simulink model "REDCS_Pipeline_IntermediateModel_FSU_29APR2022"  (R2022a)
settings: Solver=VariableStepAuto  StartTime=0.0  StopTime=3600  RelTol=1e-3
values from neighbouring files (symbols this model uses):
  Ac = (pi/4)*0.6096^2    (= 0.29186350796)    [REDCS_IntermediateModel_Parameters_29APR2022.m]
  B1 = 45    [REDCS_IntermediateModel_Parameters_29APR2022.m]
  CLOSED = 0    [REDCS_IntermediateModel_Parameters_29APR2022.m]
  EP020 = 21.9    [REDCS_IntermediateModel_Parameters_29APR2022.m]
  EP022 = 13.1    [REDCS_IntermediateModel_Parameters_29APR2022.m]
  EP024 = 54.2    [REDCS_IntermediateModel_Parameters_29APR2022.m]
  EP026 = 13.4    [REDCS_IntermediateModel_Parameters_29APR2022.m]
  EP028 = 0.5    [REDCS_IntermediateModel_Parameters_29APR2022.m]
  gamma = 1.2    [REDCS_IntermediateModel_Parameters_29APR2022.m]
  J = 5    [REDCS_IntermediateModel_Parameters_29APR2022.m]
  kf = 0.05    [REDCS_IntermediateModel_Parameters_29APR2022.m]
  Lc = 20    [REDCS_IntermediateModel_Parameters_29APR2022.m]
  OPEN = 1    [REDCS_IntermediateModel_Parameters_29APR2022.m]
  r1 = 0.05    [REDCS_IntermediateModel_Parameters_29APR2022.m]
  r2 = 0.325    [REDCS_IntermediateModel_Parameters_29APR2022.m]
  sigma = 0.90    (= 0.9)    [REDCS_IntermediateModel_Parameters_29APR2022.m]
  ValveThresh = 0.001    [REDCS_IntermediateModel_Parameters_29APR2022.m]
  ZR2000 = OPEN    (= 1)    [REDCS_IntermediateModel_Parameters_29APR2022.m]
  ZR2110 = CLOSED    (= 0)    [REDCS_IntermediateModel_Parameters_29APR2022.m]
  ZR2400 = OPEN    (= 1)    [REDCS_IntermediateModel_Parameters_29APR2022.m]
  ZR2401 = 100*OPEN    (= 100)    [REDCS_IntermediateModel_Parameters_29APR2022.m]
  ZR2510 = CLOSED    (= 0)    [REDCS_IntermediateModel_Parameters_29APR2022.m]
  ZR2600 = OPEN    (= 1)    [REDCS_IntermediateModel_Parameters_29APR2022.m]
  ZR2601 = 100*OPEN    (= 100)    [REDCS_IntermediateModel_Parameters_29APR2022.m]
  ZR2700 = OPEN    (= 1)    [REDCS_IntermediateModel_Parameters_29APR2022.m]
  ZR2701 = 100*OPEN    (= 100)    [REDCS_IntermediateModel_Parameters_29APR2022.m]
  ZR2800 = OPEN    (= 1)    [REDCS_IntermediateModel_Parameters_29APR2022.m]
  ZR2801 = 100*OPEN    (= 100)    [REDCS_IntermediateModel_Parameters_29APR2022.m]
  ZR2900 = OPEN    (= 1)    [REDCS_IntermediateModel_Parameters_29APR2022.m]
  ZR2901 = 100*OPEN    (= 100)    [REDCS_IntermediateModel_Parameters_29APR2022.m]
  ZR3900 = OPEN    (= 1)    [REDCS_IntermediateModel_Parameters_29APR2022.m]
  ZR4500 = OPEN    (= 1)    [REDCS_IntermediateModel_Parameters_29APR2022.m]
  ZR5600 = OPEN    (= 1)    [REDCS_IntermediateModel_Parameters_29APR2022.m]
  ZR7800 = CLOSED    (= 0)    [REDCS_IntermediateModel_Parameters_29APR2022.m]
undefined symbols (not defined in the file or in its folder): cotd, LEG_DEMAND_10A, LEG_DEMAND_3A, magnitude
libraries: fl_lib x170, nesl_utility x109, simulink x12, slpidlib x4
(part 2 of 4)

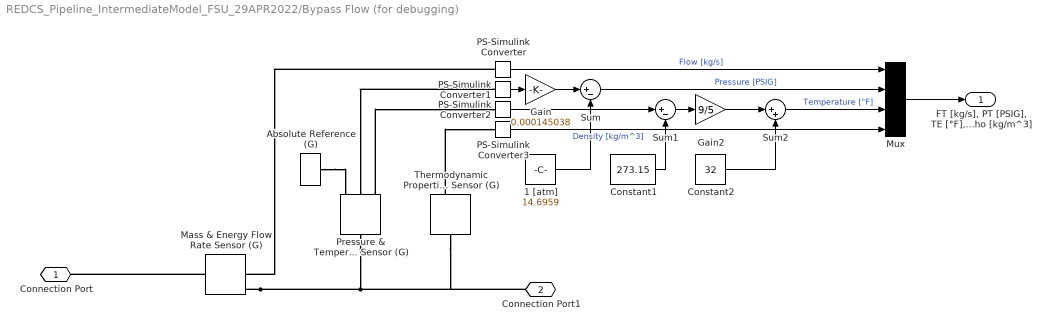
== system REDCS_Pipeline_IntermediateModel_FSU_29APR2022/Bypass Flow (for debugging) ==
  1 [atm] : Constant  Value=14.6959
  Absolute Reference (G) : fl_lib/Gas/Elements/Absolute Reference (G)
      settings: SourceProductBaseCode=PW,SS,VE  InternalSimscapePortConfiguration="{\"Bottom\":[],\"Left\":[{\"id\":\"A\",\"label\":\"\",\"type\":\"foundation.gas.gas\"}],\"Right\":[],\"Top\":[]}"
  Constant1 : Constant  Value=273.15
  Constant2 : Constant  Value=32
  Gain : Gain  Gain=0.000145038
  Gain2 : Gain  Gain=9/5
  Mass & Energy Flow Rate Sensor (G) : fl_lib/Gas/Sensors/Mass & Energy Flow Rate Sensor (G)
      settings: SourceProductBaseCode=PW,SS,VE  InternalSimscapePortConfiguration="{\"Bottom\":[],\"Left\":[{\"id\":\"A\",\"label\":\"A\",\"type\":\"foundation.gas.gas\"}],\"Right\":[{\"id\":\"B\",\"label\":\"B\",\"type\":\"foundation.gas.gas\"},{\"id\":\"M\",\"label\":\"M\",\"type\":\"output\"},{\"id\":\"PHI\",\"label\":\"Phi\",\"type\":\"output\"}],\"Top\":[]}"
  Mux : Mux
  PS-Simulink Converter{,1..3} (4 alike) : nesl_utility/PS-Simulink Converter  PhysicalDomain=network_engine_domain  SubClassName=ps_output  LeftPortType=input  RightPortType=output  PseudoPeriodic=off  Frequencies=[]  VectorFormat=1-D array  Unit=inherit  AffineConversion=off
      settings: SourceProductBaseCode=SS,PW,VE
  Pressure & Temperature Sensor (G) : fl_lib/Gas/Sensors/Pressure & Temperature Sensor (G)
      settings: SourceProductBaseCode=PW,SS,VE  InternalSimscapePortConfiguration="{\"Bottom\":[],\"Left\":[{\"id\":\"A\",\"label\":\"A\",\"type\":\"foundation.gas.gas\"}],\"Right\":[{\"id\":\"B\",\"label\":\"B\",\"type\":\"foundation.gas.gas\"},{\"id\":\"P\",\"label\":\"P\",\"type\":\"output\"},{\"id\":\"T\",\"label\":\"T\",\"type\":\"output\"}],\"Top\":[]}"
  Sum : Sum  Inputs=|+-
  Sum1 : Sum  Inputs=|+-
  Sum2 : Sum  Inputs=|++
  Thermodynamic Properties Sensor (G) : fl_lib/Gas/Sensors/Thermodynamic Properties Sensor (G)  s_std=3.8635 kJ/kg/K  p_std=0.101325 MPa  T_std=293.15 K
      settings: SourceProductBaseCode=PW,SS,VE  InternalSimscapePortConfiguration="{\"Bottom\":[],\"Left\":[{\"id\":\"A\",\"label\":\"A\",\"type\":\"foundation.gas.gas\"}],\"Right\":[{\"id\":\"H\",\"label\":\"h\",\"type\":\"output\"},{\"id\":\"RHO\",\"label\":\"rho\",\"type\":\"output\"},{\"id\":\"CP\",\"label\":\"cp\",\"type\":\"output\"},{\"id\":\"S\",\"label\":\"s\",\"type\":\"output\"}],\"Top\":[]}"
  Connection Port : PMIOPort  Side=Left
  Connection Port1 : PMIOPort  Port=2  Side=Right
  "FT [kg/s], PT [PSIG], TE [°F], rho [kg/m^3]" : Outport
  wires:
  Mux/1 -> "FT [kg/s], PT [PSIG], TE [°F], rho [kg/m^3]"/1
  PS-Simulink Converter/1 -> Mux/1  "Flow [kg/s]"
  Gain/1 -> Sum/1
  PS-Simulink Converter3/1 -> Mux/4  "Density [kg/m^3]"
  PS-Simulink Converter2/1 -> Sum1/1
  PS-Simulink Converter1/1 -> Gain/1
  1 [atm]/1 -> Sum/2
  Sum/1 -> Mux/2  "Pressure [PSIG]"
  Constant1/1 -> Sum1/2
  Sum1/1 -> Gain2/1
  Gain2/1 -> Sum2/1
  Constant2/1 -> Sum2/2
  Sum2/1 -> Mux/3  "Temperature [°F]"
  connections:
  Mass & Energy Flow Rate Sensor (G)/RConn1 -- Pressure & Temperature Sensor (G)/LConn1 -- Connection Port1/RConn1 -- Thermodynamic Properties Sensor (G)/LConn1
  Mass & Energy Flow Rate Sensor (G)/LConn1 -- Connection Port/RConn1
  PS-Simulink Converter/LConn1 -- Mass & Energy Flow Rate Sensor (G)/RConn2
  Absolute Reference (G)/LConn1 -- Pressure & Temperature Sensor (G)/RConn1
  PS-Simulink Converter1/LConn1 -- Pressure & Temperature Sensor (G)/RConn2
  Pressure & Temperature Sensor (G)/RConn3 -- PS-Simulink Converter2/LConn1
  Thermodynamic Properties Sensor (G)/RConn2 -- PS-Simulink Converter3/LConn1

== system REDCS_Pipeline_IntermediateModel_FSU_29APR2022/Check Valve ==
  Gain : Gain  Gain=1e6
  Local Restriction (G)1 : fl_lib/Gas/Elements/Local Restriction (G)  restriction_type=foundation.enum.restriction_type.variable  restriction_area=1e-3 m^2  min_area=eps m^2  max_area=(pi/4)*0.5^2-0.001 m^2  area=(pi/4)*0.5^2 m^2  Cd=1  B_lam=0.999
      settings: SourceProductBaseCode=PW,SS,VE  InternalSimscapePortConfiguration="{\"Bottom\":[],\"Left\":[{\"id\":\"A\",\"label\":\"A\",\"type\":\"foundation.gas.gas\"},{\"id\":\"area_in\",\"label\":\"AR\",\"type\":\"input\"}],\"Right\":[{\"id\":\"B\",\"label\":\"B\",\"type\":\"foundation.gas.gas\"}],\"Top\":[]}"
  Mass & Energy Flow Rate Sensor (G) : fl_lib/Gas/Sensors/Mass & Energy Flow Rate Sensor (G)
      settings: SourceProductBaseCode=PW,SS,VE  InternalSimscapePortConfiguration="{\"Bottom\":[],\"Left\":[{\"id\":\"A\",\"label\":\"A\",\"type\":\"foundation.gas.gas\"}],\"Right\":[{\"id\":\"B\",\"label\":\"B\",\"type\":\"foundation.gas.gas\"},{\"id\":\"M\",\"label\":\"M\",\"type\":\"output\"},{\"id\":\"PHI\",\"label\":\"Phi\",\"type\":\"output\"}],\"Top\":[]}"
  PS-Simulink Converter : nesl_utility/PS-Simulink Converter  PhysicalDomain=network_engine_domain  SubClassName=ps_output  LeftPortType=input  RightPortType=output  PseudoPeriodic=off  Frequencies=[]  VectorFormat=1-D array  Unit=inherit  AffineConversion=off
      settings: SourceProductBaseCode=SS,PW,VE
  Saturation : Saturate  UpperLimit=inf  LowerLimit=0  ZeroCross=off
  Sign : Signum  ZeroCross=off
  Simulink-PS Converter : nesl_utility/Simulink-PS Converter  PhysicalDomain=network_engine_domain  SubClassName=ps_input  LeftPortType=input  RightPortType=output  PseudoPeriodic=off  Frequencies=[]  NoiseDistribution=none  NoiseParameters=[]  Unit=1  AffineConversion=off  FilteringAndDerivatives=provide  SimscapeFilterOrder=1  InputFilterTimeConstant=0.001  UdotUserProvided=0
      settings: SourceProductBaseCode=SS,PW,VE
  Connection Port : PMIOPort  Side=Left
  Connection Port1 : PMIOPort  Port=2  Side=Right
  wires:
  PS-Simulink Converter/1 -> Saturation/1
  Saturation/1 -> Sign/1
  Sign/1 -> Gain/1
  Gain/1 -> Simulink-PS Converter/1
  connections:
  Simulink-PS Converter/RConn1 -- Local Restriction (G)1/LConn2
  Local Restriction (G)1/LConn1 -- Connection Port/RConn1
  Local Restriction (G)1/RConn1 -- Mass & Energy Flow Rate Sensor (G)/LConn1
  Mass & Energy Flow Rate Sensor (G)/RConn1 -- Connection Port1/RConn1
  PS-Simulink Converter/LConn1 -- Mass & Energy Flow Rate Sensor (G)/RConn2

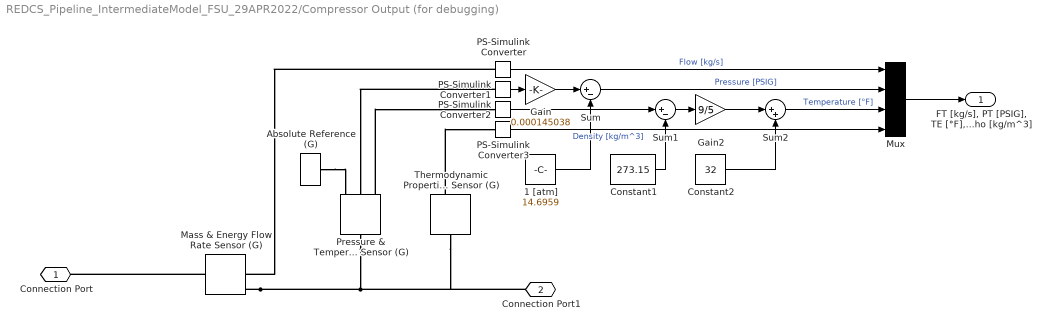
== system REDCS_Pipeline_IntermediateModel_FSU_29APR2022/Compressor Output (for debugging) ==
  1 [atm] : Constant  Value=14.6959
  Absolute Reference (G) : fl_lib/Gas/Elements/Absolute Reference (G)
      settings: SourceProductBaseCode=PW,SS,VE  InternalSimscapePortConfiguration="{\"Bottom\":[],\"Left\":[{\"id\":\"A\",\"label\":\"\",\"type\":\"foundation.gas.gas\"}],\"Right\":[],\"Top\":[]}"
  Constant1 : Constant  Value=273.15
  Constant2 : Constant  Value=32
  Gain : Gain  Gain=0.000145038
  Gain2 : Gain  Gain=9/5
  Mass & Energy Flow Rate Sensor (G) : fl_lib/Gas/Sensors/Mass & Energy Flow Rate Sensor (G)
      settings: SourceProductBaseCode=PW,SS,VE  InternalSimscapePortConfiguration="{\"Bottom\":[],\"Left\":[{\"id\":\"A\",\"label\":\"A\",\"type\":\"foundation.gas.gas\"}],\"Right\":[{\"id\":\"B\",\"label\":\"B\",\"type\":\"foundation.gas.gas\"},{\"id\":\"M\",\"label\":\"M\",\"type\":\"output\"},{\"id\":\"PHI\",\"label\":\"Phi\",\"type\":\"output\"}],\"Top\":[]}"
  Mux : Mux
  PS-Simulink Converter{,1..3} (4 alike) : nesl_utility/PS-Simulink Converter  PhysicalDomain=network_engine_domain  SubClassName=ps_output  LeftPortType=input  RightPortType=output  PseudoPeriodic=off  Frequencies=[]  VectorFormat=1-D array  Unit=inherit  AffineConversion=off
      settings: SourceProductBaseCode=SS,PW,VE
  Pressure & Temperature Sensor (G) : fl_lib/Gas/Sensors/Pressure & Temperature Sensor (G)
      settings: SourceProductBaseCode=PW,SS,VE  InternalSimscapePortConfiguration="{\"Bottom\":[],\"Left\":[{\"id\":\"A\",\"label\":\"A\",\"type\":\"foundation.gas.gas\"}],\"Right\":[{\"id\":\"B\",\"label\":\"B\",\"type\":\"foundation.gas.gas\"},{\"id\":\"P\",\"label\":\"P\",\"type\":\"output\"},{\"id\":\"T\",\"label\":\"T\",\"type\":\"output\"}],\"Top\":[]}"
  Sum : Sum  Inputs=|+-
  Sum1 : Sum  Inputs=|+-
  Sum2 : Sum  Inputs=|++
  Thermodynamic Properties Sensor (G) : fl_lib/Gas/Sensors/Thermodynamic Properties Sensor (G)  s_std=3.8635 kJ/kg/K  p_std=0.101325 MPa  T_std=293.15 K
      settings: SourceProductBaseCode=PW,SS,VE  InternalSimscapePortConfiguration="{\"Bottom\":[],\"Left\":[{\"id\":\"A\",\"label\":\"A\",\"type\":\"foundation.gas.gas\"}],\"Right\":[{\"id\":\"H\",\"label\":\"h\",\"type\":\"output\"},{\"id\":\"RHO\",\"label\":\"rho\",\"type\":\"output\"},{\"id\":\"CP\",\"label\":\"cp\",\"type\":\"output\"},{\"id\":\"S\",\"label\":\"s\",\"type\":\"output\"}],\"Top\":[]}"
  Connection Port : PMIOPort  Side=Left
  Connection Port1 : PMIOPort  Port=2  Side=Right
  "FT [kg/s], PT [PSIG], TE [°F], rho [kg/m^3]" : Outport
  wires:
  Mux/1 -> "FT [kg/s], PT [PSIG], TE [°F], rho [kg/m^3]"/1
  PS-Simulink Converter/1 -> Mux/1  "Flow [kg/s]"
  Gain/1 -> Sum/1
  PS-Simulink Converter3/1 -> Mux/4  "Density [kg/m^3]"
  PS-Simulink Converter2/1 -> Sum1/1
  PS-Simulink Converter1/1 -> Gain/1
  1 [atm]/1 -> Sum/2
  Sum/1 -> Mux/2  "Pressure [PSIG]"
  Constant1/1 -> Sum1/2
  Sum1/1 -> Gain2/1
  Gain2/1 -> Sum2/1
  Constant2/1 -> Sum2/2
  Sum2/1 -> Mux/3  "Temperature [°F]"
  connections:
  Mass & Energy Flow Rate Sensor (G)/RConn1 -- Pressure & Temperature Sensor (G)/LConn1 -- Connection Port1/RConn1 -- Thermodynamic Properties Sensor (G)/LConn1
  Mass & Energy Flow Rate Sensor (G)/LConn1 -- Connection Port/RConn1
  PS-Simulink Converter/LConn1 -- Mass & Energy Flow Rate Sensor (G)/RConn2
  Absolute Reference (G)/LConn1 -- Pressure & Temperature Sensor (G)/RConn1
  PS-Simulink Converter1/LConn1 -- Pressure & Temperature Sensor (G)/RConn2
  Pressure & Temperature Sensor (G)/RConn3 -- PS-Simulink Converter2/LConn1
  Thermodynamic Properties Sensor (G)/RConn2 -- PS-Simulink Converter3/LConn1

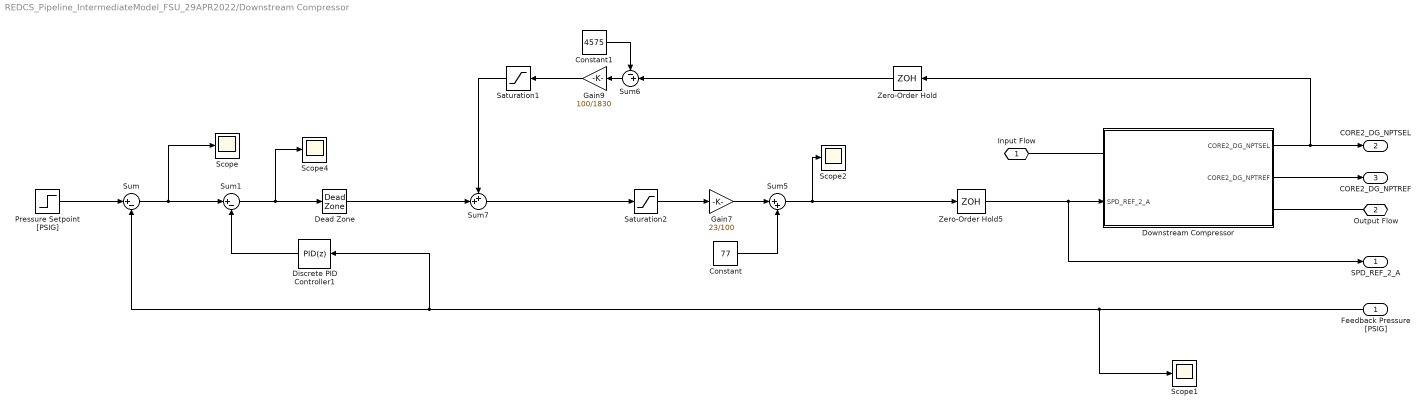
== system REDCS_Pipeline_IntermediateModel_FSU_29APR2022/Downstream Compressor ==
  Feedback Pressure [PSIG] : Inport
  Constant : Constant  Value=77
  Constant1 : Constant  Value=4575
  Dead Zone : DeadZone  LowerValue=-10  UpperValue=10
  Discrete PID Controller1 : slpidlib/PID Controller  Controller=PID  Form=Parallel  TimeDomain=Discrete-time  UseExternalTs=off  SampleTime=0.2  IntegratorMethod=Forward Euler  FilterMethod=Forward Euler  ControllerParametersSource=internal  P=0  I=0  UseKiTs=off  D=0.5  N=2  UseFilter=on  TunerSelectOption=Transfer Function Based (PID Tuner App)  InitialConditionSource=internal  InitialConditionForIntegrator=0  InitialConditionForFilter=0  DifferentiatorICPrevScaledInput=0  ExternalReset=none  TrackingMode=off  Kt=1  LimitOutput=off  SatLimitsSource=internal  UpperSaturationLimit=inf  LowerSaturationLimit=-inf  LinearizeAsGain=off  AntiWindupMode=none  Kb=1  POutMin=[]  POutMax=[]  IOutMin=[]  IOutMax=[]  DOutMin=[]  DOutMax=[]  NOutMin=[]  NOutMax=[]  SumOutMin=[]  SumOutMax=[]  SaturationOutMin=[]  SaturationOutMax=[]  PParamMin=[]  PParamMax=[]  IParamMin=[]  IParamMax=[]  DParamMin=[]  DParamMax=[]  NParamMin=[]  NParamMax=[]  KbParamMin=[]  KbParamMax=[]  KtParamMin=[]  KtParamMax=[]  KbOutMin=[]  KbOutMax=[]  KtOutMin=[]  KtOutMax=[]  IntegratorOutMin=[]  IntegratorOutMax=[]  FilterOutMin=[]  FilterOutMax=[]  SumI1OutMin=[]  SumI1OutMax=[]  SumI2OutMin=[]  SumI2OutMax=[]  SumI3OutMin=[]  SumI3OutMax=[]  SumI4OutMin=[]  SumI4OutMax=[]  SumDOutMin=[]  SumDOutMax=[]  DifferentiatorOutMin=[]  DifferentiatorOutMax=[]  FilterDiffOutCoefMin=[]  FilterDiffOutCoefMax=[]  ReciprocalOutMin=[]  ReciprocalOutMax=[]  SumDenOutMin=[]  SumDenOutMax=[]  SumNumOutMin=[]  SumNumOutMax=[]  DivideOutMin=[]  DivideOutMax=[]  UdiffTsProdOutMin=[]  UdiffTsProdOutMax=[]  NTsProdOutMin=[]  NTsProdOutMax=[]  UintegralTsProdOutMin=[]  UintegralTsProdOutMax=[]  UngainTsProdOutMin=[]  UngainTsProdOutMax=[]  IntegratorContinuousStateAttributes=''  IntegratorStateMustResolveToSignalObject=off  IntegratorRTWStateStorageClass=Auto  FilterContinuousStateAttributes=''  FilterStateMustResolveToSignalObject=off  FilterRTWStateStorageClass=Auto  ParallelPVariant=InternalParameters  IdealPVariant=Disabled  IVariant=InternalParameters  DVariant=InternalParameters  IntegratorVariant=Discrete  SatVariant=Disabled  AWVariant=Passthrough  PCopyVariant=Disabled  TRVariant=Disabled  FdbkBlocksVariant=Forward  IdealPFdbkVariant=Disabled  SatFdbkVariant=Disabled  DerivativeFilterVariant=ForwardEulerFilter  NVariant=InternalParameters  NCopyVariant=Disabled  FilterICVariant=InternalICsFilter  IntegratorICVariant=InternalICs  ExternalResetVariant=Disabled  TRSumVariant=Passthrough  SumFdbkVariant=Disabled  SumVariant=Sum_PID  TsampFilterVariant=InternalTs  TsampNgainVariant=Passthrough  TsampIntegralVariant=Passthrough  ExternalSaturationOutDataTypeStr=Inherit: Same as second input  aMode=0
  Downstream Compressor : Subsystem
      settings: PortSchema="{\"entries\":[{\"content\":{\"sides\":[{\"content\":{\"connectorIds\":[\"LConn1\",\"In1\"]},\"type\":\"ConnectorPlacement.EquallySpacedRectSide\",\"uuid\":\"0d529e09-8a6f-42a4-b3bf-cb0403a3f44f\"},{\"content\":{\"connectorIds\":[\"Out1\",\"Out2\",\"RConn1\"],\"side\":\"RIGHT\"},\"type\":\"ConnectorPlacement.EquallySpacedRectSide\",\"uuid\":\"d60f6263-f642-4388-a93f-0815d1eb49e3\"},{\"content\":{\"connectorIds\":[],\"side\":\"TOP\"},\"type\":\"ConnectorPlacement.EquallySpacedRectSide\",\"uuid\":\"9e0c1972-992e-4f26-825e-4da40d320708\"}]},\"type\":\"ConnectorPlacement.EquallySpacedConnector\",\"uuid\":\"06f6622f-0d8d-4f53-9b7f-c315a8f32589\"}],\"packageUris\":[\"http://schema.mathworks.com/mf0/Connector/R2020b\"],\"version\":\"1.0\"}"
  Gain7 : Gain  Gain=23/100
  Gain9 : Gain  Gain=100/1830
  Pressure Setpoint [PSIG] : Step  Time=720  Before=LEG_DEMAND_10A(1)  After=LEG_DEMAND_10A(2)  SampleTime=0
  Saturation1 : Saturate  UpperLimit=100  LowerLimit=0
  Saturation2 : Saturate  UpperLimit=100  LowerLimit=0
  Scope{,1..2,4} (4 alike) : Scope
  Sum : Sum  Inputs=|+-
  Sum1 : Sum  Inputs=|+-
  Sum5 : Sum  Inputs=|++
  Sum6 : Sum  Inputs=-+|
  Sum7 : Sum  Inputs=++|
  Zero-Order Hold : ZeroOrderHold  SampleTime=0.2
  Zero-Order Hold5 : ZeroOrderHold  SampleTime=0.2
  Input Flow : PMIOPort  Side=Left
  Output Flow : PMIOPort  Port=2  Side=Right
  SPD_REF_2_A : Outport
  CORE2_DG_NPTSEL : Outport  Port=2
  CORE2_DG_NPTREF : Outport  Port=3
  wires:
  Sum7/1 -> Saturation2/1
  Feedback Pressure [PSIG]/1 -> Discrete PID Controller1/1, Sum/2, Scope1/1
  Zero-Order Hold5/1 -> Downstream Compressor/1(SPD_REF_2_A), SPD_REF_2_A/1
  Sum5/1 -> Scope2/1, Zero-Order Hold5/1
  Zero-Order Hold/1 -> Sum6/2
  Constant1/1 -> Sum6/1
  Sum/1 -> Scope/1, Sum1/1
  Gain9/1 -> Saturation1/1
  Constant/1 -> Sum5/2
  Saturation2/1 -> Gain7/1
  Gain7/1 -> Sum5/1
  Sum6/1 -> Gain9/1
  Pressure Setpoint [PSIG]/1 -> Sum/1
  Discrete PID Controller1/1 -> Sum1/2
  Saturation1/1 -> Sum7/1
  Sum1/1 -> Dead Zone/1, Scope4/1
  Downstream Compressor/1(CORE2_DG_NPTSEL) -> CORE2_DG_NPTSEL/1, Zero-Order Hold/1
  Dead Zone/1 -> Sum7/2
  Downstream Compressor/2(CORE2_DG_NPTREF) -> CORE2_DG_NPTREF/1
  connections:
  Output Flow/RConn1 -- Downstream Compressor/RConn1
  Downstream Compressor/LConn1 -- Input Flow/RConn1

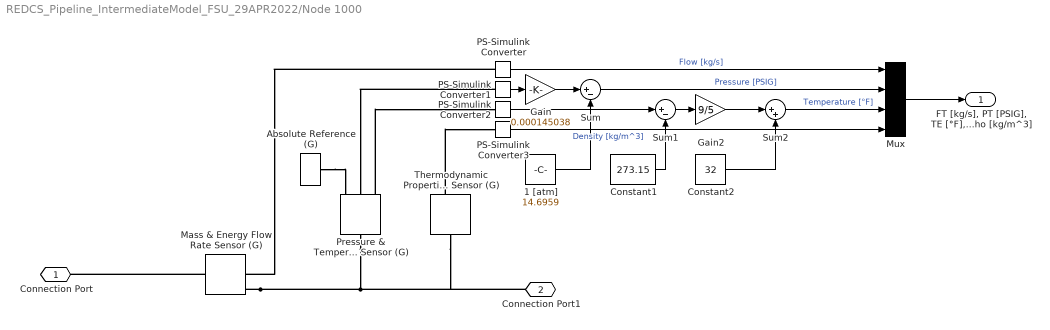
== system REDCS_Pipeline_IntermediateModel_FSU_29APR2022/Node 1000 ==
  1 [atm] : Constant  Value=14.6959
  Absolute Reference (G) : fl_lib/Gas/Elements/Absolute Reference (G)
      settings: SourceProductBaseCode=PW,SS,VE  InternalSimscapePortConfiguration="{\"Bottom\":[],\"Left\":[{\"id\":\"A\",\"label\":\"\",\"type\":\"foundation.gas.gas\"}],\"Right\":[],\"Top\":[]}"
  Constant1 : Constant  Value=273.15
  Constant2 : Constant  Value=32
  Gain : Gain  Gain=0.000145038
  Gain2 : Gain  Gain=9/5
  Mass & Energy Flow Rate Sensor (G) : fl_lib/Gas/Sensors/Mass & Energy Flow Rate Sensor (G)
      settings: SourceProductBaseCode=PW,SS,VE  InternalSimscapePortConfiguration="{\"Bottom\":[],\"Left\":[{\"id\":\"A\",\"label\":\"A\",\"type\":\"foundation.gas.gas\"}],\"Right\":[{\"id\":\"B\",\"label\":\"B\",\"type\":\"foundation.gas.gas\"},{\"id\":\"M\",\"label\":\"M\",\"type\":\"output\"},{\"id\":\"PHI\",\"label\":\"Phi\",\"type\":\"output\"}],\"Top\":[]}"
  Mux : Mux
  PS-Simulink Converter{,1..3} (4 alike) : nesl_utility/PS-Simulink Converter  PhysicalDomain=network_engine_domain  SubClassName=ps_output  LeftPortType=input  RightPortType=output  PseudoPeriodic=off  Frequencies=[]  VectorFormat=1-D array  Unit=inherit  AffineConversion=off
      settings: SourceProductBaseCode=SS,PW,VE
  Pressure & Temperature Sensor (G) : fl_lib/Gas/Sensors/Pressure & Temperature Sensor (G)
      settings: SourceProductBaseCode=PW,SS,VE  InternalSimscapePortConfiguration="{\"Bottom\":[],\"Left\":[{\"id\":\"A\",\"label\":\"A\",\"type\":\"foundation.gas.gas\"}],\"Right\":[{\"id\":\"B\",\"label\":\"B\",\"type\":\"foundation.gas.gas\"},{\"id\":\"P\",\"label\":\"P\",\"type\":\"output\"},{\"id\":\"T\",\"label\":\"T\",\"type\":\"output\"}],\"Top\":[]}"
  Sum : Sum  Inputs=|+-
  Sum1 : Sum  Inputs=|+-
  Sum2 : Sum  Inputs=|++
  Thermodynamic Properties Sensor (G) : fl_lib/Gas/Sensors/Thermodynamic Properties Sensor (G)  s_std=3.8635 kJ/kg/K  p_std=0.101325 MPa  T_std=293.15 K
      settings: SourceProductBaseCode=PW,SS,VE  InternalSimscapePortConfiguration="{\"Bottom\":[],\"Left\":[{\"id\":\"A\",\"label\":\"A\",\"type\":\"foundation.gas.gas\"}],\"Right\":[{\"id\":\"H\",\"label\":\"h\",\"type\":\"output\"},{\"id\":\"RHO\",\"label\":\"rho\",\"type\":\"output\"},{\"id\":\"CP\",\"label\":\"cp\",\"type\":\"output\"},{\"id\":\"S\",\"label\":\"s\",\"type\":\"output\"}],\"Top\":[]}"
  Connection Port : PMIOPort  Side=Left
  Connection Port1 : PMIOPort  Port=2  Side=Right
  "FT [kg/s], PT [PSIG], TE [°F], rho [kg/m^3]" : Outport
  wires:
  Mux/1 -> "FT [kg/s], PT [PSIG], TE [°F], rho [kg/m^3]"/1
  PS-Simulink Converter/1 -> Mux/1  "Flow [kg/s]"
  Gain/1 -> Sum/1
  PS-Simulink Converter3/1 -> Mux/4  "Density [kg/m^3]"
  PS-Simulink Converter2/1 -> Sum1/1
  PS-Simulink Converter1/1 -> Gain/1
  1 [atm]/1 -> Sum/2
  Sum/1 -> Mux/2  "Pressure [PSIG]"
  Constant1/1 -> Sum1/2
  Sum1/1 -> Gain2/1
  Gain2/1 -> Sum2/1
  Constant2/1 -> Sum2/2
  Sum2/1 -> Mux/3  "Temperature [°F]"
  connections:
  Mass & Energy Flow Rate Sensor (G)/RConn1 -- Pressure & Temperature Sensor (G)/LConn1 -- Connection Port1/RConn1 -- Thermodynamic Properties Sensor (G)/LConn1
  Mass & Energy Flow Rate Sensor (G)/LConn1 -- Connection Port/RConn1
  PS-Simulink Converter/LConn1 -- Mass & Energy Flow Rate Sensor (G)/RConn2
  Absolute Reference (G)/LConn1 -- Pressure & Temperature Sensor (G)/RConn1
  PS-Simulink Converter1/LConn1 -- Pressure & Temperature Sensor (G)/RConn2
  Pressure & Temperature Sensor (G)/RConn3 -- PS-Simulink Converter2/LConn1
  Thermodynamic Properties Sensor (G)/RConn2 -- PS-Simulink Converter3/LConn1

== system REDCS_Pipeline_IntermediateModel_FSU_29APR2022/Node 2000 ==
  1 [atm] : Constant  Value=14.6959
  Absolute Reference (G) : fl_lib/Gas/Elements/Absolute Reference (G)
      settings: SourceProductBaseCode=PW,SS,VE  InternalSimscapePortConfiguration="{\"Bottom\":[],\"Left\":[{\"id\":\"A\",\"label\":\"\",\"type\":\"foundation.gas.gas\"}],\"Right\":[],\"Top\":[]}"
  Constant1 : Constant  Value=273.15
  Constant2 : Constant  Value=32
  Gain : Gain  Gain=0.000145038
  Gain2 : Gain  Gain=9/5
  Mass & Energy Flow Rate Sensor (G) : fl_lib/Gas/Sensors/Mass & Energy Flow Rate Sensor (G)
      settings: SourceProductBaseCode=PW,SS,VE  InternalSimscapePortConfiguration="{\"Bottom\":[],\"Left\":[{\"id\":\"A\",\"label\":\"A\",\"type\":\"foundation.gas.gas\"}],\"Right\":[{\"id\":\"B\",\"label\":\"B\",\"type\":\"foundation.gas.gas\"},{\"id\":\"M\",\"label\":\"M\",\"type\":\"output\"},{\"id\":\"PHI\",\"label\":\"Phi\",\"type\":\"output\"}],\"Top\":[]}"
  Mux : Mux
  PS-Simulink Converter{,1..3} (4 alike) : nesl_utility/PS-Simulink Converter  PhysicalDomain=network_engine_domain  SubClassName=ps_output  LeftPortType=input  RightPortType=output  PseudoPeriodic=off  Frequencies=[]  VectorFormat=1-D array  Unit=inherit  AffineConversion=off
      settings: SourceProductBaseCode=SS,PW,VE
  Pressure & Temperature Sensor (G) : fl_lib/Gas/Sensors/Pressure & Temperature Sensor (G)
      settings: SourceProductBaseCode=PW,SS,VE  InternalSimscapePortConfiguration="{\"Bottom\":[],\"Left\":[{\"id\":\"A\",\"label\":\"A\",\"type\":\"foundation.gas.gas\"}],\"Right\":[{\"id\":\"B\",\"label\":\"B\",\"type\":\"foundation.gas.gas\"},{\"id\":\"P\",\"label\":\"P\",\"type\":\"output\"},{\"id\":\"T\",\"label\":\"T\",\"type\":\"output\"}],\"Top\":[]}"
  Sum : Sum  Inputs=|+-
  Sum1 : Sum  Inputs=|+-
  Sum2 : Sum  Inputs=|++
  Thermodynamic Properties Sensor (G) : fl_lib/Gas/Sensors/Thermodynamic Properties Sensor (G)  s_std=3.8635 kJ/kg/K  p_std=0.101325 MPa  T_std=293.15 K
      settings: SourceProductBaseCode=PW,SS,VE  InternalSimscapePortConfiguration="{\"Bottom\":[],\"Left\":[{\"id\":\"A\",\"label\":\"A\",\"type\":\"foundation.gas.gas\"}],\"Right\":[{\"id\":\"H\",\"label\":\"h\",\"type\":\"output\"},{\"id\":\"RHO\",\"label\":\"rho\",\"type\":\"output\"},{\"id\":\"CP\",\"label\":\"cp\",\"type\":\"output\"},{\"id\":\"S\",\"label\":\"s\",\"type\":\"output\"}],\"Top\":[]}"
  Connection Port : PMIOPort  Side=Left
  Connection Port1 : PMIOPort  Port=2  Side=Right
  "FT [kg/s], PT [PSIG], TE [°F], rho [kg/m^3]" : Outport
  wires:
  Mux/1 -> "FT [kg/s], PT [PSIG], TE [°F], rho [kg/m^3]"/1
  PS-Simulink Converter/1 -> Mux/1  "Flow [kg/s]"
  Gain/1 -> Sum/1
  PS-Simulink Converter3/1 -> Mux/4  "Density [kg/m^3]"
  PS-Simulink Converter2/1 -> Sum1/1
  PS-Simulink Converter1/1 -> Gain/1
  1 [atm]/1 -> Sum/2
  Sum/1 -> Mux/2  "Pressure [PSIG]"
  Constant1/1 -> Sum1/2
  Sum1/1 -> Gain2/1
  Gain2/1 -> Sum2/1
  Constant2/1 -> Sum2/2
  Sum2/1 -> Mux/3  "Temperature [°F]"
  connections:
  Mass & Energy Flow Rate Sensor (G)/RConn1 -- Pressure & Temperature Sensor (G)/LConn1 -- Connection Port1/RConn1 -- Thermodynamic Properties Sensor (G)/LConn1
  Mass & Energy Flow Rate Sensor (G)/LConn1 -- Connection Port/RConn1
  PS-Simulink Converter/LConn1 -- Mass & Energy Flow Rate Sensor (G)/RConn2
  Absolute Reference (G)/LConn1 -- Pressure & Temperature Sensor (G)/RConn1
  PS-Simulink Converter1/LConn1 -- Pressure & Temperature Sensor (G)/RConn2
  Pressure & Temperature Sensor (G)/RConn3 -- PS-Simulink Converter2/LConn1
  Thermodynamic Properties Sensor (G)/RConn2 -- PS-Simulink Converter3/LConn1

== system REDCS_Pipeline_IntermediateModel_FSU_29APR2022/Node 2100 ==
  1 [atm] : Constant  Value=14.6959
  Absolute Reference (G) : fl_lib/Gas/Elements/Absolute Reference (G)
      settings: SourceProductBaseCode=PW,SS,VE  InternalSimscapePortConfiguration="{\"Bottom\":[],\"Left\":[{\"id\":\"A\",\"label\":\"\",\"type\":\"foundation.gas.gas\"}],\"Right\":[],\"Top\":[]}"
  Constant1 : Constant  Value=273.15
  Constant2 : Constant  Value=32
  Gain : Gain  Gain=0.000145038
  Gain2 : Gain  Gain=9/5
  Mass & Energy Flow Rate Sensor (G) : fl_lib/Gas/Sensors/Mass & Energy Flow Rate Sensor (G)
      settings: SourceProductBaseCode=PW,SS,VE  InternalSimscapePortConfiguration="{\"Bottom\":[],\"Left\":[{\"id\":\"A\",\"label\":\"A\",\"type\":\"foundation.gas.gas\"}],\"Right\":[{\"id\":\"B\",\"label\":\"B\",\"type\":\"foundation.gas.gas\"},{\"id\":\"M\",\"label\":\"M\",\"type\":\"output\"},{\"id\":\"PHI\",\"label\":\"Phi\",\"type\":\"output\"}],\"Top\":[]}"
  Mux : Mux
  PS-Simulink Converter{,1..3} (4 alike) : nesl_utility/PS-Simulink Converter  PhysicalDomain=network_engine_domain  SubClassName=ps_output  LeftPortType=input  RightPortType=output  PseudoPeriodic=off  Frequencies=[]  VectorFormat=1-D array  Unit=inherit  AffineConversion=off
      settings: SourceProductBaseCode=SS,PW,VE
  Pressure & Temperature Sensor (G) : fl_lib/Gas/Sensors/Pressure & Temperature Sensor (G)
      settings: SourceProductBaseCode=PW,SS,VE  InternalSimscapePortConfiguration="{\"Bottom\":[],\"Left\":[{\"id\":\"A\",\"label\":\"A\",\"type\":\"foundation.gas.gas\"}],\"Right\":[{\"id\":\"B\",\"label\":\"B\",\"type\":\"foundation.gas.gas\"},{\"id\":\"P\",\"label\":\"P\",\"type\":\"output\"},{\"id\":\"T\",\"label\":\"T\",\"type\":\"output\"}],\"Top\":[]}"
  Sum : Sum  Inputs=|+-
  Sum1 : Sum  Inputs=|+-
  Sum2 : Sum  Inputs=|++
  Thermodynamic Properties Sensor (G) : fl_lib/Gas/Sensors/Thermodynamic Properties Sensor (G)  s_std=3.8635 kJ/kg/K  p_std=0.101325 MPa  T_std=293.15 K
      settings: SourceProductBaseCode=PW,SS,VE  InternalSimscapePortConfiguration="{\"Bottom\":[],\"Left\":[{\"id\":\"A\",\"label\":\"A\",\"type\":\"foundation.gas.gas\"}],\"Right\":[{\"id\":\"H\",\"label\":\"h\",\"type\":\"output\"},{\"id\":\"RHO\",\"label\":\"rho\",\"type\":\"output\"},{\"id\":\"CP\",\"label\":\"cp\",\"type\":\"output\"},{\"id\":\"S\",\"label\":\"s\",\"type\":\"output\"}],\"Top\":[]}"
  Connection Port : PMIOPort  Side=Left
  Connection Port1 : PMIOPort  Port=2  Side=Right
  "FT [kg/s], PT [PSIG], TE [°F], rho [kg/m^3]" : Outport
  wires:
  Mux/1 -> "FT [kg/s], PT [PSIG], TE [°F], rho [kg/m^3]"/1
  PS-Simulink Converter/1 -> Mux/1  "Flow [kg/s]"
  Gain/1 -> Sum/1
  PS-Simulink Converter3/1 -> Mux/4  "Density [kg/m^3]"
  PS-Simulink Converter2/1 -> Sum1/1
  PS-Simulink Converter1/1 -> Gain/1
  1 [atm]/1 -> Sum/2
  Sum/1 -> Mux/2  "Pressure [PSIG]"
  Constant1/1 -> Sum1/2
  Sum1/1 -> Gain2/1
  Gain2/1 -> Sum2/1
  Constant2/1 -> Sum2/2
  Sum2/1 -> Mux/3  "Temperature [°F]"
  connections:
  Mass & Energy Flow Rate Sensor (G)/RConn1 -- Pressure & Temperature Sensor (G)/LConn1 -- Connection Port1/RConn1 -- Thermodynamic Properties Sensor (G)/LConn1
  Mass & Energy Flow Rate Sensor (G)/LConn1 -- Connection Port/RConn1
  PS-Simulink Converter/LConn1 -- Mass & Energy Flow Rate Sensor (G)/RConn2
  Absolute Reference (G)/LConn1 -- Pressure & Temperature Sensor (G)/RConn1
  PS-Simulink Converter1/LConn1 -- Pressure & Temperature Sensor (G)/RConn2
  Pressure & Temperature Sensor (G)/RConn3 -- PS-Simulink Converter2/LConn1
  Thermodynamic Properties Sensor (G)/RConn2 -- PS-Simulink Converter3/LConn1

== system REDCS_Pipeline_IntermediateModel_FSU_29APR2022/Node 2200 ==
  1 [atm] : Constant  Value=14.6959
  Absolute Reference (G) : fl_lib/Gas/Elements/Absolute Reference (G)
      settings: SourceProductBaseCode=PW,SS,VE  InternalSimscapePortConfiguration="{\"Bottom\":[],\"Left\":[{\"id\":\"A\",\"label\":\"\",\"type\":\"foundation.gas.gas\"}],\"Right\":[],\"Top\":[]}"
  Constant1 : Constant  Value=273.15
  Constant2 : Constant  Value=32
  Gain : Gain  Gain=0.000145038
  Gain2 : Gain  Gain=9/5
  Mass & Energy Flow Rate Sensor (G) : fl_lib/Gas/Sensors/Mass & Energy Flow Rate Sensor (G)
      settings: SourceProductBaseCode=PW,SS,VE  InternalSimscapePortConfiguration="{\"Bottom\":[],\"Left\":[{\"id\":\"A\",\"label\":\"A\",\"type\":\"foundation.gas.gas\"}],\"Right\":[{\"id\":\"B\",\"label\":\"B\",\"type\":\"foundation.gas.gas\"},{\"id\":\"M\",\"label\":\"M\",\"type\":\"output\"},{\"id\":\"PHI\",\"label\":\"Phi\",\"type\":\"output\"}],\"Top\":[]}"
  Mux : Mux
  PS-Simulink Converter{,1..3} (4 alike) : nesl_utility/PS-Simulink Converter  PhysicalDomain=network_engine_domain  SubClassName=ps_output  LeftPortType=input  RightPortType=output  PseudoPeriodic=off  Frequencies=[]  VectorFormat=1-D array  Unit=inherit  AffineConversion=off
      settings: SourceProductBaseCode=SS,PW,VE
  Pressure & Temperature Sensor (G) : fl_lib/Gas/Sensors/Pressure & Temperature Sensor (G)
      settings: SourceProductBaseCode=PW,SS,VE  InternalSimscapePortConfiguration="{\"Bottom\":[],\"Left\":[{\"id\":\"A\",\"label\":\"A\",\"type\":\"foundation.gas.gas\"}],\"Right\":[{\"id\":\"B\",\"label\":\"B\",\"type\":\"foundation.gas.gas\"},{\"id\":\"P\",\"label\":\"P\",\"type\":\"output\"},{\"id\":\"T\",\"label\":\"T\",\"type\":\"output\"}],\"Top\":[]}"
  Sum : Sum  Inputs=|+-
  Sum1 : Sum  Inputs=|+-
  Sum2 : Sum  Inputs=|++
  Thermodynamic Properties Sensor (G) : fl_lib/Gas/Sensors/Thermodynamic Properties Sensor (G)  s_std=3.8635 kJ/kg/K  p_std=0.101325 MPa  T_std=293.15 K
      settings: SourceProductBaseCode=PW,SS,VE  InternalSimscapePortConfiguration="{\"Bottom\":[],\"Left\":[{\"id\":\"A\",\"label\":\"A\",\"type\":\"foundation.gas.gas\"}],\"Right\":[{\"id\":\"H\",\"label\":\"h\",\"type\":\"output\"},{\"id\":\"RHO\",\"label\":\"rho\",\"type\":\"output\"},{\"id\":\"CP\",\"label\":\"cp\",\"type\":\"output\"},{\"id\":\"S\",\"label\":\"s\",\"type\":\"output\"}],\"Top\":[]}"
  Connection Port : PMIOPort  Side=Left
  Connection Port1 : PMIOPort  Port=2  Side=Right
  "FT [kg/s], PT [PSIG], TE [°F], rho [kg/m^3]" : Outport
  wires:
  Mux/1 -> "FT [kg/s], PT [PSIG], TE [°F], rho [kg/m^3]"/1
  PS-Simulink Converter/1 -> Mux/1  "Flow [kg/s]"
  Gain/1 -> Sum/1
  PS-Simulink Converter3/1 -> Mux/4  "Density [kg/m^3]"
  PS-Simulink Converter2/1 -> Sum1/1
  PS-Simulink Converter1/1 -> Gain/1
  1 [atm]/1 -> Sum/2
  Sum/1 -> Mux/2  "Pressure [PSIG]"
  Constant1/1 -> Sum1/2
  Sum1/1 -> Gain2/1
  Gain2/1 -> Sum2/1
  Constant2/1 -> Sum2/2
  Sum2/1 -> Mux/3  "Temperature [°F]"
  connections:
  Mass & Energy Flow Rate Sensor (G)/RConn1 -- Pressure & Temperature Sensor (G)/LConn1 -- Connection Port1/RConn1 -- Thermodynamic Properties Sensor (G)/LConn1
  Mass & Energy Flow Rate Sensor (G)/LConn1 -- Connection Port/RConn1
  PS-Simulink Converter/LConn1 -- Mass & Energy Flow Rate Sensor (G)/RConn2
  Absolute Reference (G)/LConn1 -- Pressure & Temperature Sensor (G)/RConn1
  PS-Simulink Converter1/LConn1 -- Pressure & Temperature Sensor (G)/RConn2
  Pressure & Temperature Sensor (G)/RConn3 -- PS-Simulink Converter2/LConn1
  Thermodynamic Properties Sensor (G)/RConn2 -- PS-Simulink Converter3/LConn1

== system REDCS_Pipeline_IntermediateModel_FSU_29APR2022/Node 2300 ==
  1 [atm] : Constant  Value=14.6959
  Absolute Reference (G) : fl_lib/Gas/Elements/Absolute Reference (G)
      settings: SourceProductBaseCode=PW,SS,VE  InternalSimscapePortConfiguration="{\"Bottom\":[],\"Left\":[{\"id\":\"A\",\"label\":\"\",\"type\":\"foundation.gas.gas\"}],\"Right\":[],\"Top\":[]}"
  Constant1 : Constant  Value=273.15
  Constant2 : Constant  Value=32
  Gain : Gain  Gain=0.000145038
  Gain2 : Gain  Gain=9/5
  Mass & Energy Flow Rate Sensor (G) : fl_lib/Gas/Sensors/Mass & Energy Flow Rate Sensor (G)
      settings: SourceProductBaseCode=PW,SS,VE  InternalSimscapePortConfiguration="{\"Bottom\":[],\"Left\":[{\"id\":\"A\",\"label\":\"A\",\"type\":\"foundation.gas.gas\"}],\"Right\":[{\"id\":\"B\",\"label\":\"B\",\"type\":\"foundation.gas.gas\"},{\"id\":\"M\",\"label\":\"M\",\"type\":\"output\"},{\"id\":\"PHI\",\"label\":\"Phi\",\"type\":\"output\"}],\"Top\":[]}"
  Mux : Mux
  PS-Simulink Converter{,1..3} (4 alike) : nesl_utility/PS-Simulink Converter  PhysicalDomain=network_engine_domain  SubClassName=ps_output  LeftPortType=input  RightPortType=output  PseudoPeriodic=off  Frequencies=[]  VectorFormat=1-D array  Unit=inherit  AffineConversion=off
      settings: SourceProductBaseCode=SS,PW,VE
  Pressure & Temperature Sensor (G) : fl_lib/Gas/Sensors/Pressure & Temperature Sensor (G)
      settings: SourceProductBaseCode=PW,SS,VE  InternalSimscapePortConfiguration="{\"Bottom\":[],\"Left\":[{\"id\":\"A\",\"label\":\"A\",\"type\":\"foundation.gas.gas\"}],\"Right\":[{\"id\":\"B\",\"label\":\"B\",\"type\":\"foundation.gas.gas\"},{\"id\":\"P\",\"label\":\"P\",\"type\":\"output\"},{\"id\":\"T\",\"label\":\"T\",\"type\":\"output\"}],\"Top\":[]}"
  Sum : Sum  Inputs=|+-
  Sum1 : Sum  Inputs=|+-
  Sum2 : Sum  Inputs=|++
  Thermodynamic Properties Sensor (G) : fl_lib/Gas/Sensors/Thermodynamic Properties Sensor (G)  s_std=3.8635 kJ/kg/K  p_std=0.101325 MPa  T_std=293.15 K
      settings: SourceProductBaseCode=PW,SS,VE  InternalSimscapePortConfiguration="{\"Bottom\":[],\"Left\":[{\"id\":\"A\",\"label\":\"A\",\"type\":\"foundation.gas.gas\"}],\"Right\":[{\"id\":\"H\",\"label\":\"h\",\"type\":\"output\"},{\"id\":\"RHO\",\"label\":\"rho\",\"type\":\"output\"},{\"id\":\"CP\",\"label\":\"cp\",\"type\":\"output\"},{\"id\":\"S\",\"label\":\"s\",\"type\":\"output\"}],\"Top\":[]}"
  Connection Port : PMIOPort  Side=Left
  Connection Port1 : PMIOPort  Port=2  Side=Right
  "FT [kg/s], PT [PSIG], TE [°F], rho [kg/m^3]" : Outport
  wires:
  Mux/1 -> "FT [kg/s], PT [PSIG], TE [°F], rho [kg/m^3]"/1
  PS-Simulink Converter/1 -> Mux/1  "Flow [kg/s]"
  Gain/1 -> Sum/1
  PS-Simulink Converter3/1 -> Mux/4  "Density [kg/m^3]"
  PS-Simulink Converter2/1 -> Sum1/1
  PS-Simulink Converter1/1 -> Gain/1
  1 [atm]/1 -> Sum/2
  Sum/1 -> Mux/2  "Pressure [PSIG]"
  Constant1/1 -> Sum1/2
  Sum1/1 -> Gain2/1
  Gain2/1 -> Sum2/1
  Constant2/1 -> Sum2/2
  Sum2/1 -> Mux/3  "Temperature [°F]"
  connections:
  Mass & Energy Flow Rate Sensor (G)/RConn1 -- Pressure & Temperature Sensor (G)/LConn1 -- Connection Port1/RConn1 -- Thermodynamic Properties Sensor (G)/LConn1
  Mass & Energy Flow Rate Sensor (G)/LConn1 -- Connection Port/RConn1
  PS-Simulink Converter/LConn1 -- Mass & Energy Flow Rate Sensor (G)/RConn2
  Absolute Reference (G)/LConn1 -- Pressure & Temperature Sensor (G)/RConn1
  PS-Simulink Converter1/LConn1 -- Pressure & Temperature Sensor (G)/RConn2
  Pressure & Temperature Sensor (G)/RConn3 -- PS-Simulink Converter2/LConn1
  Thermodynamic Properties Sensor (G)/RConn2 -- PS-Simulink Converter3/LConn1

== system REDCS_Pipeline_IntermediateModel_FSU_29APR2022/Node 2301 ==
  1 [atm] : Constant  Value=14.6959
  Absolute Reference (G) : fl_lib/Gas/Elements/Absolute Reference (G)
      settings: SourceProductBaseCode=PW,SS,VE  InternalSimscapePortConfiguration="{\"Bottom\":[],\"Left\":[{\"id\":\"A\",\"label\":\"\",\"type\":\"foundation.gas.gas\"}],\"Right\":[],\"Top\":[]}"
  Constant1 : Constant  Value=273.15
  Constant2 : Constant  Value=32
  Gain : Gain  Gain=0.000145038
  Gain2 : Gain  Gain=9/5
  Mass & Energy Flow Rate Sensor (G) : fl_lib/Gas/Sensors/Mass & Energy Flow Rate Sensor (G)
      settings: SourceProductBaseCode=PW,SS,VE  InternalSimscapePortConfiguration="{\"Bottom\":[],\"Left\":[{\"id\":\"A\",\"label\":\"A\",\"type\":\"foundation.gas.gas\"}],\"Right\":[{\"id\":\"B\",\"label\":\"B\",\"type\":\"foundation.gas.gas\"},{\"id\":\"M\",\"label\":\"M\",\"type\":\"output\"},{\"id\":\"PHI\",\"label\":\"Phi\",\"type\":\"output\"}],\"Top\":[]}"
  Mux : Mux
  PS-Simulink Converter{,1..3} (4 alike) : nesl_utility/PS-Simulink Converter  PhysicalDomain=network_engine_domain  SubClassName=ps_output  LeftPortType=input  RightPortType=output  PseudoPeriodic=off  Frequencies=[]  VectorFormat=1-D array  Unit=inherit  AffineConversion=off
      settings: SourceProductBaseCode=SS,PW,VE
  Pressure & Temperature Sensor (G) : fl_lib/Gas/Sensors/Pressure & Temperature Sensor (G)
      settings: SourceProductBaseCode=PW,SS,VE  InternalSimscapePortConfiguration="{\"Bottom\":[],\"Left\":[{\"id\":\"A\",\"label\":\"A\",\"type\":\"foundation.gas.gas\"}],\"Right\":[{\"id\":\"B\",\"label\":\"B\",\"type\":\"foundation.gas.gas\"},{\"id\":\"P\",\"label\":\"P\",\"type\":\"output\"},{\"id\":\"T\",\"label\":\"T\",\"type\":\"output\"}],\"Top\":[]}"
  Sum : Sum  Inputs=|+-
  Sum1 : Sum  Inputs=|+-
  Sum2 : Sum  Inputs=|++
  Thermodynamic Properties Sensor (G) : fl_lib/Gas/Sensors/Thermodynamic Properties Sensor (G)  s_std=3.8635 kJ/kg/K  p_std=0.101325 MPa  T_std=293.15 K
      settings: SourceProductBaseCode=PW,SS,VE  InternalSimscapePortConfiguration="{\"Bottom\":[],\"Left\":[{\"id\":\"A\",\"label\":\"A\",\"type\":\"foundation.gas.gas\"}],\"Right\":[{\"id\":\"H\",\"label\":\"h\",\"type\":\"output\"},{\"id\":\"RHO\",\"label\":\"rho\",\"type\":\"output\"},{\"id\":\"CP\",\"label\":\"cp\",\"type\":\"output\"},{\"id\":\"S\",\"label\":\"s\",\"type\":\"output\"}],\"Top\":[]}"
  Connection Port : PMIOPort  Side=Left
  Connection Port1 : PMIOPort  Port=2  Side=Right
  "FT [kg/s], PT [PSIG], TE [°F], rho [kg/m^3]" : Outport
  wires:
  Mux/1 -> "FT [kg/s], PT [PSIG], TE [°F], rho [kg/m^3]"/1
  PS-Simulink Converter/1 -> Mux/1  "Flow [kg/s]"
  Gain/1 -> Sum/1
  PS-Simulink Converter3/1 -> Mux/4  "Density [kg/m^3]"
  PS-Simulink Converter2/1 -> Sum1/1
  PS-Simulink Converter1/1 -> Gain/1
  1 [atm]/1 -> Sum/2
  Sum/1 -> Mux/2  "Pressure [PSIG]"
  Constant1/1 -> Sum1/2
  Sum1/1 -> Gain2/1
  Gain2/1 -> Sum2/1
  Constant2/1 -> Sum2/2
  Sum2/1 -> Mux/3  "Temperature [°F]"
  connections:
  Mass & Energy Flow Rate Sensor (G)/RConn1 -- Pressure & Temperature Sensor (G)/LConn1 -- Connection Port1/RConn1 -- Thermodynamic Properties Sensor (G)/LConn1
  Mass & Energy Flow Rate Sensor (G)/LConn1 -- Connection Port/RConn1
  PS-Simulink Converter/LConn1 -- Mass & Energy Flow Rate Sensor (G)/RConn2
  Absolute Reference (G)/LConn1 -- Pressure & Temperature Sensor (G)/RConn1
  PS-Simulink Converter1/LConn1 -- Pressure & Temperature Sensor (G)/RConn2
  Pressure & Temperature Sensor (G)/RConn3 -- PS-Simulink Converter2/LConn1
  Thermodynamic Properties Sensor (G)/RConn2 -- PS-Simulink Converter3/LConn1

== system REDCS_Pipeline_IntermediateModel_FSU_29APR2022/Node 2350 ==
  1 [atm] : Constant  Value=14.6959
  Absolute Reference (G) : fl_lib/Gas/Elements/Absolute Reference (G)
      settings: SourceProductBaseCode=PW,SS,VE  InternalSimscapePortConfiguration="{\"Bottom\":[],\"Left\":[{\"id\":\"A\",\"label\":\"\",\"type\":\"foundation.gas.gas\"}],\"Right\":[],\"Top\":[]}"
  Constant1 : Constant  Value=273.15
  Constant2 : Constant  Value=32
  Gain : Gain  Gain=0.000145038
  Gain2 : Gain  Gain=9/5
  Mass & Energy Flow Rate Sensor (G) : fl_lib/Gas/Sensors/Mass & Energy Flow Rate Sensor (G)
      settings: SourceProductBaseCode=PW,SS,VE  InternalSimscapePortConfiguration="{\"Bottom\":[],\"Left\":[{\"id\":\"A\",\"label\":\"A\",\"type\":\"foundation.gas.gas\"}],\"Right\":[{\"id\":\"B\",\"label\":\"B\",\"type\":\"foundation.gas.gas\"},{\"id\":\"M\",\"label\":\"M\",\"type\":\"output\"},{\"id\":\"PHI\",\"label\":\"Phi\",\"type\":\"output\"}],\"Top\":[]}"
  Mux : Mux
  PS-Simulink Converter{,1..3} (4 alike) : nesl_utility/PS-Simulink Converter  PhysicalDomain=network_engine_domain  SubClassName=ps_output  LeftPortType=input  RightPortType=output  PseudoPeriodic=off  Frequencies=[]  VectorFormat=1-D array  Unit=inherit  AffineConversion=off
      settings: SourceProductBaseCode=SS,PW,VE
  Pressure & Temperature Sensor (G) : fl_lib/Gas/Sensors/Pressure & Temperature Sensor (G)
      settings: SourceProductBaseCode=PW,SS,VE  InternalSimscapePortConfiguration="{\"Bottom\":[],\"Left\":[{\"id\":\"A\",\"label\":\"A\",\"type\":\"foundation.gas.gas\"}],\"Right\":[{\"id\":\"B\",\"label\":\"B\",\"type\":\"foundation.gas.gas\"},{\"id\":\"P\",\"label\":\"P\",\"type\":\"output\"},{\"id\":\"T\",\"label\":\"T\",\"type\":\"output\"}],\"Top\":[]}"
  Sum : Sum  Inputs=|+-
  Sum1 : Sum  Inputs=|+-
  Sum2 : Sum  Inputs=|++
  Thermodynamic Properties Sensor (G) : fl_lib/Gas/Sensors/Thermodynamic Properties Sensor (G)  s_std=3.8635 kJ/kg/K  p_std=0.101325 MPa  T_std=293.15 K
      settings: SourceProductBaseCode=PW,SS,VE  InternalSimscapePortConfiguration="{\"Bottom\":[],\"Left\":[{\"id\":\"A\",\"label\":\"A\",\"type\":\"foundation.gas.gas\"}],\"Right\":[{\"id\":\"H\",\"label\":\"h\",\"type\":\"output\"},{\"id\":\"RHO\",\"label\":\"rho\",\"type\":\"output\"},{\"id\":\"CP\",\"label\":\"cp\",\"type\":\"output\"},{\"id\":\"S\",\"label\":\"s\",\"type\":\"output\"}],\"Top\":[]}"
  Connection Port : PMIOPort  Side=Left
  Connection Port1 : PMIOPort  Port=2  Side=Right
  "FT [kg/s], PT [PSIG], TE [°F], rho [kg/m^3]" : Outport
  wires:
  Mux/1 -> "FT [kg/s], PT [PSIG], TE [°F], rho [kg/m^3]"/1
  PS-Simulink Converter/1 -> Mux/1  "Flow [kg/s]"
  Gain/1 -> Sum/1
  PS-Simulink Converter3/1 -> Mux/4  "Density [kg/m^3]"
  PS-Simulink Converter2/1 -> Sum1/1
  PS-Simulink Converter1/1 -> Gain/1
  1 [atm]/1 -> Sum/2
  Sum/1 -> Mux/2  "Pressure [PSIG]"
  Constant1/1 -> Sum1/2
  Sum1/1 -> Gain2/1
  Gain2/1 -> Sum2/1
  Constant2/1 -> Sum2/2
  Sum2/1 -> Mux/3  "Temperature [°F]"
  connections:
  Mass & Energy Flow Rate Sensor (G)/RConn1 -- Pressure & Temperature Sensor (G)/LConn1 -- Connection Port1/RConn1 -- Thermodynamic Properties Sensor (G)/LConn1
  Mass & Energy Flow Rate Sensor (G)/LConn1 -- Connection Port/RConn1
  PS-Simulink Converter/LConn1 -- Mass & Energy Flow Rate Sensor (G)/RConn2
  Absolute Reference (G)/LConn1 -- Pressure & Temperature Sensor (G)/RConn1
  PS-Simulink Converter1/LConn1 -- Pressure & Temperature Sensor (G)/RConn2
  Pressure & Temperature Sensor (G)/RConn3 -- PS-Simulink Converter2/LConn1
  Thermodynamic Properties Sensor (G)/RConn2 -- PS-Simulink Converter3/LConn1

== system REDCS_Pipeline_IntermediateModel_FSU_29APR2022/Node 2400 ==
  1 [atm] : Constant  Value=14.6959
  Absolute Reference (G) : fl_lib/Gas/Elements/Absolute Reference (G)
      settings: SourceProductBaseCode=PW,SS,VE  InternalSimscapePortConfiguration="{\"Bottom\":[],\"Left\":[{\"id\":\"A\",\"label\":\"\",\"type\":\"foundation.gas.gas\"}],\"Right\":[],\"Top\":[]}"
  Constant1 : Constant  Value=273.15
  Constant2 : Constant  Value=32
  Gain : Gain  Gain=0.000145038
  Gain2 : Gain  Gain=9/5
  Mass & Energy Flow Rate Sensor (G) : fl_lib/Gas/Sensors/Mass & Energy Flow Rate Sensor (G)
      settings: SourceProductBaseCode=PW,SS,VE  InternalSimscapePortConfiguration="{\"Bottom\":[],\"Left\":[{\"id\":\"A\",\"label\":\"A\",\"type\":\"foundation.gas.gas\"}],\"Right\":[{\"id\":\"B\",\"label\":\"B\",\"type\":\"foundation.gas.gas\"},{\"id\":\"M\",\"label\":\"M\",\"type\":\"output\"},{\"id\":\"PHI\",\"label\":\"Phi\",\"type\":\"output\"}],\"Top\":[]}"
  Mux : Mux
  PS-Simulink Converter{,1..3} (4 alike) : nesl_utility/PS-Simulink Converter  PhysicalDomain=network_engine_domain  SubClassName=ps_output  LeftPortType=input  RightPortType=output  PseudoPeriodic=off  Frequencies=[]  VectorFormat=1-D array  Unit=inherit  AffineConversion=off
      settings: SourceProductBaseCode=SS,PW,VE
  Pressure & Temperature Sensor (G) : fl_lib/Gas/Sensors/Pressure & Temperature Sensor (G)
      settings: SourceProductBaseCode=PW,SS,VE  InternalSimscapePortConfiguration="{\"Bottom\":[],\"Left\":[{\"id\":\"A\",\"label\":\"A\",\"type\":\"foundation.gas.gas\"}],\"Right\":[{\"id\":\"B\",\"label\":\"B\",\"type\":\"foundation.gas.gas\"},{\"id\":\"P\",\"label\":\"P\",\"type\":\"output\"},{\"id\":\"T\",\"label\":\"T\",\"type\":\"output\"}],\"Top\":[]}"
  Sum : Sum  Inputs=|+-
  Sum1 : Sum  Inputs=|+-
  Sum2 : Sum  Inputs=|++
  Thermodynamic Properties Sensor (G) : fl_lib/Gas/Sensors/Thermodynamic Properties Sensor (G)  s_std=3.8635 kJ/kg/K  p_std=0.101325 MPa  T_std=293.15 K
      settings: SourceProductBaseCode=PW,SS,VE  InternalSimscapePortConfiguration="{\"Bottom\":[],\"Left\":[{\"id\":\"A\",\"label\":\"A\",\"type\":\"foundation.gas.gas\"}],\"Right\":[{\"id\":\"H\",\"label\":\"h\",\"type\":\"output\"},{\"id\":\"RHO\",\"label\":\"rho\",\"type\":\"output\"},{\"id\":\"CP\",\"label\":\"cp\",\"type\":\"output\"},{\"id\":\"S\",\"label\":\"s\",\"type\":\"output\"}],\"Top\":[]}"
  Connection Port : PMIOPort  Side=Left
  Connection Port1 : PMIOPort  Port=2  Side=Right
  "FT [kg/s], PT [PSIG], TE [°F], rho [kg/m^3]" : Outport
  wires:
  Mux/1 -> "FT [kg/s], PT [PSIG], TE [°F], rho [kg/m^3]"/1
  PS-Simulink Converter/1 -> Mux/1  "Flow [kg/s]"
  Gain/1 -> Sum/1
  PS-Simulink Converter3/1 -> Mux/4  "Density [kg/m^3]"
  PS-Simulink Converter2/1 -> Sum1/1
  PS-Simulink Converter1/1 -> Gain/1
  1 [atm]/1 -> Sum/2
  Sum/1 -> Mux/2  "Pressure [PSIG]"
  Constant1/1 -> Sum1/2
  Sum1/1 -> Gain2/1
  Gain2/1 -> Sum2/1
  Constant2/1 -> Sum2/2
  Sum2/1 -> Mux/3  "Temperature [°F]"
  connections:
  Mass & Energy Flow Rate Sensor (G)/RConn1 -- Pressure & Temperature Sensor (G)/LConn1 -- Connection Port1/RConn1 -- Thermodynamic Properties Sensor (G)/LConn1
  Mass & Energy Flow Rate Sensor (G)/LConn1 -- Connection Port/RConn1
  PS-Simulink Converter/LConn1 -- Mass & Energy Flow Rate Sensor (G)/RConn2
  Absolute Reference (G)/LConn1 -- Pressure & Temperature Sensor (G)/RConn1
  PS-Simulink Converter1/LConn1 -- Pressure & Temperature Sensor (G)/RConn2
  Pressure & Temperature Sensor (G)/RConn3 -- PS-Simulink Converter2/LConn1
  Thermodynamic Properties Sensor (G)/RConn2 -- PS-Simulink Converter3/LConn1
